simulink library "NeuroMuscularLibrary"  (R2019b)
settings: Solver=ode45  StartTime=0.0  StopTime=10.0  RelTol=1e-3  EnableMultiTasking=on
values from neighbouring files (symbols this model uses):
  a_18_19 = 116    [Prosthesis3R60Params.m]
  a_18_21 = 34    [Prosthesis3R60Params.m]
  a_2_3 = 18    [Prosthesis3R60Params.m]
  angle_offset = 0    [Prosthesis3R60Params.m]
  ankle_height = 0.08    [BodyMechParams.m]
  c = 0.05    [BodyMechParams.m]
  c_jointstop = 0.3 / (pi/180)    (= 17.1887338539)    [BodyMechParams.m]
  c_stance_comp_a0 = 885.0653    [Prosthesis3R60Params.m]
  c_stance_comp_a1 = 2.1443    [Prosthesis3R60Params.m]
  cg14 = 1/2*L14    (= 0.0475)    [Prosthesis3R60Params.m]
  cg25 = (5.45/11.05)*L25    (= 0.0379527149321)    [Prosthesis3R60Params.m]
  cg3 = (3.6/10.4)*L3    (= 0.0306346153846)    [Prosthesis3R60Params.m]
  d_fBall = 0.1    [BodyMechParams.m]
  d_fHeel = 0.05    [BodyMechParams.m]
  deltaLegAngleThr = 8*pi/180    (= 0.13962634016)    [CMGParams.m]
  DeltaThRef = 2e-3    (= 0.002)    [BodyMechParams.m]
  dt_visual = 0.001    [Prosthesis3R60Params.m]
  eref = 0.04    [BodyMechParams.m]
  Fmax = 4000    [MuscleEnergyTest.m]
  FmaxGLU = 1500    [BodyMechParams.m]
  footBallToAnkleDist = 0.16    [BodyMechParams.m]
  footBallToCenterDist = footLength/2    (= 0.1)    [BodyMechParams.m]
  footBallToHeelDist = footLength    (= 0.2)    [BodyMechParams.m]
  footCenterToCGDist = 0.14 - footBallToCenterDist    (= 0.04)    [BodyMechParams.m]
  footInertia = 0.005    [BodyMechParams.m]
  footLength = 0.2    [BodyMechParams.m]
  footMass = 1.25    [BodyMechParams.m]
  FT = 20    [MuscleEnergyTest.m]
  FT_GLU = 47.6    [BodyMechParams.m]
  g = 9.80665    [BodyMechParams.m]
  groundTheta = [atan(diff(groundZ)./diff(groundX)), 0]    [generateGround.m]
  groundZ = groundZ * stepSize/(largestStep+eps)    [generateGround.m]
  hatCenterToCGDist = 0.35 - hatHipToCenterDistLen    (= -0.05)    [BodyMechParams.m]
  hatHipToCenterDistLen = hatLength/2    (= 0.4)    [BodyMechParams.m]
  hatInertia = 3    [BodyMechParams.m]
  hatLeftHipToCenterDistWidth = .15    (= 0.15)    [BodyMechParams.m]
  hatLength = 0.8    [BodyMechParams.m]
  hatMass = 53.5    [BodyMechParams.m]
  hatThickness = 0.2    [BodyMechParams.m]
  hatWidth = 0.4    [BodyMechParams.m]
  J1011 = (4130)*1e-9    (= 4.13e-06)    [Prosthesis3R60Params.m]
  J1415 = (1.18*1e5)*1e-9    (= 0.000118)    [Prosthesis3R60Params.m]
  J18192021 = (6.86*1e4)*1e-9    (= 6.86e-05)    [Prosthesis3R60Params.m]
  J2526 = (3.59*1e4)*1e-9    (= 3.59e-05)    [Prosthesis3R60Params.m]
  J3467 = (25.96*1e4)*1e-9    (= 0.0002596)    [Prosthesis3R60Params.m]
  K = 5    [BodyMechParams.m]
  k_gn = k_gn/2    (= 39226.6)    [BodyMechParams.m]
  k_gt = k_gt/2    (= 39226.6)    [BodyMechParams.m]
  k_pressure = hatMass * g / DeltaThRef    (= 262327.8875)    [BodyMechParams.m]
  k_stance = 130000    [Prosthesis3R60Params.m]
  k_swing = 18750    [Prosthesis3R60Params.m]
  L0_stance = 0.08925    [Prosthesis3R60Params.m]
  L0_swing = 0.0896    [Prosthesis3R60Params.m]
  L10 = 7.9*1e-3    (= 0.0079)    [Prosthesis3R60Params.m]
  L11 = 3.3*1e-3    (= 0.0033)    [Prosthesis3R60Params.m]
  L14 = 95*1e-3    (= 0.095)    [Prosthesis3R60Params.m]
  L15 = 8.2*1e-3    (= 0.0082)    [Prosthesis3R60Params.m]
  L18 = 25.1*1e-3    (= 0.0251)    [Prosthesis3R60Params.m]
  L19 = 17.7*1e-3    (= 0.0177)    [Prosthesis3R60Params.m]
  L20 = 26*1e-3    (= 0.026)    [Prosthesis3R60Params.m]
  L21 = 1.7*1e-3    (= 0.0017)    [Prosthesis3R60Params.m]
  L25 = 76.95*1e-3    (= 0.07695)    [Prosthesis3R60Params.m]
  L26 = 2.8*1e-3    (= 0.0028)    [Prosthesis3R60Params.m]
  L3 = 88.5*1e-3    (= 0.0885)    [Prosthesis3R60Params.m]
  L4 = 1.7*1e-3    (= 0.0017)    [Prosthesis3R60Params.m]
  L6 = 40.25*1e-3    (= 0.04025)    [Prosthesis3R60Params.m]
  L7 = 14.9*1e-3    (= 0.0149)    [Prosthesis3R60Params.m]
  leg_l = [(thighLength - ankle_height/2) (shankLength - ankle_height/2)]    [BodyMechParams.m]
  legAngleSpeedMax = 10    [CMGParams.m]
  lopt = 0.055    [MuscleEnergyTest.m]
  loptBFSH = 0.12    [BodyMechParams.m]
  loptGAS = 0.05    [BodyMechParams.m]
  loptGLU = 0.11    [BodyMechParams.m]
  loptHAB = 0.09    [BodyMechParams.m]
  loptHAD = 0.10    (= 0.1)    [BodyMechParams.m]
  loptHAM = 0.10    (= 0.1)    [BodyMechParams.m]
  loptHFL = 0.11    [BodyMechParams.m]
  loptRF = 0.08    [BodyMechParams.m]
  loptSOL = 0.04    [BodyMechParams.m]
  loptTA = 0.06    [BodyMechParams.m]
  loptVAS = 0.08    [BodyMechParams.m]
  lslack = 0.245    [MuscleEnergyTest.m]
  lslackBFSH = 0.10    (= 0.1)    [BodyMechParams.m]
  lslackGAS = 0.40    (= 0.4)    [BodyMechParams.m]
  lslackGLU = 0.13    [BodyMechParams.m]
  lslackHAB = 0.07    [BodyMechParams.m]
  lslackHAD = 0.18    [BodyMechParams.m]
  lslackHAM = 0.31    [BodyMechParams.m]
  lslackHFL = 0.10    (= 0.1)    [BodyMechParams.m]
  lslackRF = 0.35    [BodyMechParams.m]
  lslackSOL = 0.26    [BodyMechParams.m]
  lslackTA = 0.24    [BodyMechParams.m]
  lslackVAS = 0.23    [BodyMechParams.m]
  m1011 = 49.5*1e-3    (= 0.0495)    [Prosthesis3R60Params.m]
  m1415 = 123.8*1e-3    (= 0.1238)    [Prosthesis3R60Params.m]
  m18192021 = 196.6*1e-3    (= 0.1966)    [Prosthesis3R60Params.m]
  m2526 = 58.3*1e-3    (= 0.0583)    [Prosthesis3R60Params.m]
  m3467 = 253.3*1e-3    (= 0.2533)    [Prosthesis3R60Params.m]
  mu_slide = 0.8    [BodyMechParams.m]
  mu_stick = 0.9    [BodyMechParams.m]
  N = 1.5    [BodyMechParams.m]    (also in cmaes.m = size(x,1); mergeCompareEnergyCosts.m = {S.name})
  phiKneeUpLimit = 5*pi/180    (= 0.0872664625997)    [BodyMechParams.m]
  phimaxGASa = (100-90)*pi/180    (= 0.174532925199)    [BodyMechParams.m]
  phimaxGASk = (180-140)*pi/180    (= 0.698131700798)    [BodyMechParams.m]
  phimaxRFk = (180-165)*pi/180    (= 0.261799387799)    [BodyMechParams.m]
  phimaxSOL = (100-90)*pi/180    (= 0.174532925199)    [BodyMechParams.m]
  phimaxTA = (80-90)*pi/180    (= -0.174532925199)    [BodyMechParams.m]
  phimaxVAS = (180-165)*pi/180    (= 0.261799387799)    [BodyMechParams.m]
  phirefBFSH = (180-160)*pi/180    (= 0.349065850399)    [BodyMechParams.m]
  phirefGASa = (80-90)*pi/180    (= -0.174532925199)    [BodyMechParams.m]
  phirefGASk = (180-165)*pi/180    (= 0.261799387799)    [BodyMechParams.m]
  phirefGLU = (120-180)*pi/180    (= -1.0471975512)    [BodyMechParams.m]
  phirefHAB = 10*pi/180    (= 0.174532925199)    [BodyMechParams.m]
  phirefHAD = 15*pi/180    (= 0.261799387799)    [BodyMechParams.m]
  phirefHAMh = (150-180)*pi/180    (= -0.523598775598)    [BodyMechParams.m]
  phirefHAMk = (180-180)*pi/180    (= 0)    [BodyMechParams.m]
  phirefHFL = (160-180)*pi/180    (= -0.349065850399)    [BodyMechParams.m]
  phirefRFh = (170-180)*pi/180    (= -0.174532925199)    [BodyMechParams.m]
  phirefRFk = (180-125)*pi/180    (= 0.959931088597)    [BodyMechParams.m]
  phirefSOL = (90-90)*pi/180    (= 0)    [BodyMechParams.m]
  ... (+64 more)
undefined symbols (not defined in the file or in its folder): ankleBackDriveGain, ankleCJointstop, ankleDgain, ankleFilterPID, ankleFilterSEA, ankleGearEff, ankleGearRatio, ankleIgain, ankleInitialAngle, ankleInputMass, ankleIntCoulomb, ankleIntDamping, ankleIntStatic, ankleParallelSpringDamping, ankleParallelSpringOffset, ankleParallelSpringStiffness, anklePgain, anklePlantarLimit, ankleSEADamping, ankleSEAStiffness, ankleTendonMass, ankleWMaxJointstop, D12_F, D12_S, D12_T, D12z_T, D13_F, D1G_F, D1G_HAT, D1G_S, D1G_T, D1Gy_F, DeltaS, DeltaSGLU, DeltaSHFL, dryFrictionDamping, dryFrictionStiffness, dryFrictionVelThresh, footMassp, FourBarL1, FourBarL3, GainDphiHATGLUst, GainDphiHATHABst, GainDphiHATHADst, GainDphiHATHFLst, GainFGASst, GainFGLUst, GainFHABst, GainFHAMst, GainFSOLst, GainFSOLTAst, GainFVASst, GainGAS, GainGLU, GainGLUswing, GainHAM, GainHAMHFL ... (+194)
libraries: sm_lib x332, nesl_utility x156, simulink x33, dspswit3 x30, $bdroot x19, simulink_extras x7
(part 3 of 15)

== system NeuroMuscularLibrary/HATs ==
  Brick Solid : sm_lib/Body Elements/Brick Solid  GraphicAmbientColor=[0.15 0.15 0.15 1.0]  BasedOnType=Mass  BrickDimensions=[L_HAT 0.1 2*D12z_T]  BrickDimensionUnits=m  CenterOfMass=[0 0 0]  CenterOfMassUnits=m  GraphicDiffuseColor=[0.5 0.5 0.5]  Density=0  DensityUnits=kg/m^3  DoExposeReferenceFrame=on  GraphicEmissiveColor=[0.0 0.0 0.0 1.0]  ExportEntireGeometry=off  SerializedFrames=<Frames/>  MarkerShape=Sphere  MarkerSize=10  GraphicType=FromGeometry  InertiaType=CalculateFromGeometry  Mass=0  MassUnits=kg  MomentsOfInertia=[1 1 1]  MomentsOfInertiaUnits=kg*m^2  GraphicOpacity=1.0  ProductsOfInertia=[0 0 0]  ProductsOfInertiaUnits=kg*m^2  GraphicShininess=75  GraphicSpecularColor=[0.5 0.5 0.5 1.0]  GraphicVisPropType=SimpleVisualProperties
  CS4 : sm_lib/Frames and Transforms/Rigid Transform  TranslationMethod=Cartesian  TranslationStandardOffset=0  TranslationLengthUnit=m  TranslationStandardAxis=+Z  TranslationCartesianOffset=[0 0 2*D12z_T]  TranslationROffset=0  TranslationROffsetUnits=m  TranslationZOffset=0  TranslationZOffsetUnits=m  TranslationThetaOffset=0  TranslationThetaOffsetUnits=deg  RotationMethod=None  RotationAngleUnits=deg  RotationStandardAxis=+Z  RotationAngle=0.0  RotationArbitraryAxis=[0 0 1]  FollAlignAxisA=+X  BaseAlignAxisA=+Y  FollAlignAxisB=+Y  BaseAlignAxisB=+Z  RotationSequenceAxes=FollowerAxes  RotationSequence=XYX  RotationSequenceAngles=[0 0 0]  RotationSequenceAnglesUnits=deg  RotationMatrix=[1 0 0; 0 1 0; 0 0 1]
  Inertia : sm_lib/Body Elements/Inertia  InertiaType=Custom  Mass=m_HAT  MassUnits=kg  CenterOfMass=[0 0 0]  CenterOfMassUnits=m  MomentsOfInertia="[Inx_HAT Iny_HAT  In_HAT]"  MomentsOfInertiaUnits=kg*m^2  ProductsOfInertia=[0 0 0]  ProductsOfInertiaUnits=kg*m^2  GraphicType=None  MarkerShape=Inertia  MarkerSize=20  GraphicVisPropType=SimpleVisualProperties  GraphicDiffuseColor=[0.5 0.5 0.5]  GraphicSpecularColor=[0.5 0.5 0.5 1.0]  GraphicAmbientColor=[0.15 0.15 0.15 1.0]  GraphicEmissiveColor=[0.0 0.0 0.0 1.0]  GraphicShininess=75  GraphicOpacity=1.0
  Mux{,1..5} (6 alike) : Mux  Inputs=3
  PS-Simulink Converter{,1..8} (9 alike) : nesl_utility/PS-Simulink Converter  PhysicalDomain=network_engine_domain  SubClassName=ps_output  LeftPortType=input  RightPortType=output  PseudoPeriodic=off  Frequencies=[]  Unit=m  AffineConversion=off
  PS-Simulink Converter{9..17} (9 alike) : nesl_utility/PS-Simulink Converter  PhysicalDomain=network_engine_domain  SubClassName=ps_output  LeftPortType=input  RightPortType=output  PseudoPeriodic=off  Frequencies=[]  Unit=m/s  AffineConversion=off
  Reference Frame : sm_lib/Frames and Transforms/Reference Frame
  TO: X-forward Y-up Z-lateral : sm_lib/Frames and Transforms/Rigid Transform  TranslationMethod=StandardAxis  TranslationStandardOffset=1*D12z_T/2  TranslationLengthUnit=m  TranslationStandardAxis=+Y  TranslationCartesianOffset=[0 0 0]  TranslationROffset=0  TranslationROffsetUnits=m  TranslationZOffset=0  TranslationZOffsetUnits=m  TranslationThetaOffset=0  TranslationThetaOffsetUnits=deg  RotationMethod=AlignedAxes  RotationAngleUnits=deg  RotationStandardAxis=+Z  RotationAngle=0  RotationArbitraryAxis=[0 0 1]  FollAlignAxisA=+Y  BaseAlignAxisA=+Z  FollAlignAxisB=+X  BaseAlignAxisB=+X  RotationSequenceAxes=FollowerAxes  RotationSequence=XYX  RotationSequenceAngles=[0 0 0]  RotationSequenceAnglesUnits=deg  RotationMatrix=[1 0 0; 0 1 0; 0 0 1]
  To CG : sm_lib/Frames and Transforms/Rigid Transform  TranslationMethod=Cartesian  TranslationStandardOffset=0  TranslationLengthUnit=m  TranslationStandardAxis=+Z  TranslationCartesianOffset=[D1G_HAT 0 D12z_T]  TranslationROffset=0  TranslationROffsetUnits=m  TranslationZOffset=0  TranslationZOffsetUnits=m  TranslationThetaOffset=0  TranslationThetaOffsetUnits=deg  RotationMethod=None  RotationAngleUnits=deg  RotationStandardAxis=+Z  RotationAngle=0.0  RotationArbitraryAxis=[0 0 1]  FollAlignAxisA=+X  BaseAlignAxisA=+Y  FollAlignAxisB=+Y  BaseAlignAxisB=+Z  RotationSequenceAxes=FollowerAxes  RotationSequence=XYX  RotationSequenceAngles=[0 0 0]  RotationSequenceAnglesUnits=deg  RotationMatrix=[1 0 0; 0 1 0; 0 0 1]
  To center : sm_lib/Frames and Transforms/Rigid Transform  TranslationMethod=Cartesian  TranslationStandardOffset=0  TranslationLengthUnit=m  TranslationStandardAxis=+Z  TranslationCartesianOffset=[L_HAT/2 0 D12z_T]  TranslationROffset=0  TranslationROffsetUnits=m  TranslationZOffset=0  TranslationZOffsetUnits=m  TranslationThetaOffset=0  TranslationThetaOffsetUnits=deg  RotationMethod=None  RotationAngleUnits=deg  RotationStandardAxis=+Z  RotationAngle=0.0  RotationArbitraryAxis=[0 0 1]  FollAlignAxisA=+Z  BaseAlignAxisA=-X  FollAlignAxisB=+Y  BaseAlignAxisB=+Y  RotationSequenceAxes=FollowerAxes  RotationSequence=XYX  RotationSequenceAngles=[0 0 0]  RotationSequenceAnglesUnits=deg  RotationMatrix=[1 0 0; 0 1 0; 0 0 1]
  Transform Sensor : sm_lib/Frames and Transforms/Transform Sensor  MeasurementFrame=NonRotatingBase  SenseAngle=off  SenseAxis=off  SenseAngle1=off  SenseAngle2=off  SenseAngle3=off  SenseQ=off  SenseR=off  SenseOmegaX=off  SenseOmegaY=off  SenseOmegaZ=off  SenseOmega1=off  SenseOmega2=off  SenseOmega3=off  SenseQDot=off  SenseRDot=off  SenseAlphaX=off  SenseAlphaY=off  SenseAlphaZ=off  SenseAlpha1=off  SenseAlpha2=off  SenseAlpha3=off  SenseQDDot=off  SenseRDDot=off  SenseX=on  SenseY=on  SenseZ=on  SenseRad=off  SenseAzim=off  SenseDist=off  SenseInc=off  SenseXDot=on  SenseYDot=on  SenseZDot=on  SenseRadDot=off  SenseAzimDot=off  SenseDistDot=off  SenseIncDot=off  SenseXDDot=off  SenseYDDot=off  SenseZDDot=off  SenseRadDDot=off  SenseAzimDDot=off  SenseDistDDot=off  SenseIncDDot=off
  Transform Sensor1 : sm_lib/Frames and Transforms/Transform Sensor  MeasurementFrame=NonRotatingBase  SenseAngle=off  SenseAxis=off  SenseAngle1=off  SenseAngle2=off  SenseAngle3=off  SenseQ=off  SenseR=off  SenseOmegaX=off  SenseOmegaY=off  SenseOmegaZ=off  SenseOmega1=off  SenseOmega2=off  SenseOmega3=off  SenseQDot=off  SenseRDot=off  SenseAlphaX=off  SenseAlphaY=off  SenseAlphaZ=off  SenseAlpha1=off  SenseAlpha2=off  SenseAlpha3=off  SenseQDDot=off  SenseRDDot=off  SenseX=on  SenseY=on  SenseZ=on  SenseRad=off  SenseAzim=off  SenseDist=off  SenseInc=off  SenseXDot=on  SenseYDot=on  SenseZDot=on  SenseRadDot=off  SenseAzimDot=off  SenseDistDot=off  SenseIncDot=off  SenseXDDot=off  SenseYDDot=off  SenseZDDot=off  SenseRadDDot=off  SenseAzimDDot=off  SenseDistDDot=off  SenseIncDDot=off
  Transform Sensor2 : sm_lib/Frames and Transforms/Transform Sensor  MeasurementFrame=NonRotatingBase  SenseAngle=off  SenseAxis=off  SenseAngle1=off  SenseAngle2=off  SenseAngle3=off  SenseQ=off  SenseR=off  SenseOmegaX=off  SenseOmegaY=off  SenseOmegaZ=off  SenseOmega1=off  SenseOmega2=off  SenseOmega3=off  SenseQDot=off  SenseRDot=off  SenseAlphaX=off  SenseAlphaY=off  SenseAlphaZ=off  SenseAlpha1=off  SenseAlpha2=off  SenseAlpha3=off  SenseQDDot=off  SenseRDDot=off  SenseX=on  SenseY=on  SenseZ=on  SenseRad=off  SenseAzim=off  SenseDist=off  SenseInc=off  SenseXDot=on  SenseYDot=on  SenseZDot=on  SenseRadDot=off  SenseAzimDot=off  SenseDistDot=off  SenseIncDot=off  SenseXDDot=off  SenseYDDot=off  SenseZDDot=off  SenseRadDDot=off  SenseAzimDDot=off  SenseDistDDot=off  SenseIncDDot=off
  World Frame1 : sm_lib/Frames and Transforms/World Frame
  Left hip : PMIOPort  Side=Left
  Right hip : PMIOPort  Port=2  Side=Left
  CG : PMIOPort  Port=3  Side=Right
  Left hip pos : Outport
  Left hip vel : Outport  Port=2
  HAT  pos : Outport  Port=3
  HAT  vel : Outport  Port=4
  Right hip pos : Outport  Port=5
  Right hip vel : Outport  Port=6
  wires:
  Mux/1 -> HAT  pos/1
  PS-Simulink Converter1/1 -> Mux/3
  PS-Simulink Converter2/1 -> Mux/2
  PS-Simulink Converter/1 -> Mux/1
  PS-Simulink Converter3/1 -> Mux1/1
  PS-Simulink Converter4/1 -> Mux1/2
  PS-Simulink Converter5/1 -> Mux1/3
  Mux2/1 -> Right hip pos/1
  PS-Simulink Converter8/1 -> Mux2/3
  PS-Simulink Converter7/1 -> Mux2/2
  PS-Simulink Converter6/1 -> Mux2/1
  Mux5/1 -> HAT  vel/1
  PS-Simulink Converter9/1 -> Mux5/1
  PS-Simulink Converter10/1 -> Mux5/2
  PS-Simulink Converter11/1 -> Mux5/3
  PS-Simulink Converter12/1 -> Mux3/1
  PS-Simulink Converter13/1 -> Mux3/2
  PS-Simulink Converter14/1 -> Mux3/3
  Mux3/1 -> Left hip vel/1
  PS-Simulink Converter15/1 -> Mux4/1
  PS-Simulink Converter16/1 -> Mux4/2
  PS-Simulink Converter17/1 -> Mux4/3
  Mux4/1 -> Right hip vel/1
  Mux1/1 -> Left hip pos/1
  connections:
  Reference Frame/RConn1 -- TO: X-forward Y-up Z-lateral/RConn1 -- Transform Sensor/LConn1 -- Transform Sensor2/LConn1 -- Transform Sensor1/LConn1
  Transform Sensor/RConn4 -- PS-Simulink Converter1/LConn1
  Transform Sensor/RConn3 -- PS-Simulink Converter2/LConn1
  PS-Simulink Converter/LConn1 -- Transform Sensor/RConn2
  Left hip/RConn1 -- Transform Sensor1/RConn1 -- CS4/LConn1 -- To CG/LConn1 -- To center/LConn1
  To CG/RConn1 -- CG/RConn1 -- Transform Sensor/RConn1 -- Inertia/RConn1
  Brick Solid/RConn1 -- To center/RConn1
  Right hip/RConn1 -- Transform Sensor2/RConn1 -- CS4/RConn1
  Transform Sensor1/RConn2 -- PS-Simulink Converter3/LConn1
  Transform Sensor1/RConn3 -- PS-Simulink Converter4/LConn1
  Transform Sensor1/RConn4 -- PS-Simulink Converter5/LConn1
  Transform Sensor2/RConn4 -- PS-Simulink Converter8/LConn1
  Transform Sensor2/RConn3 -- PS-Simulink Converter7/LConn1
  Transform Sensor2/RConn2 -- PS-Simulink Converter6/LConn1
  Transform Sensor/RConn7 -- PS-Simulink Converter11/LConn1
  Transform Sensor/RConn6 -- PS-Simulink Converter10/LConn1
  Transform Sensor/RConn5 -- PS-Simulink Converter9/LConn1
  Transform Sensor1/RConn5 -- PS-Simulink Converter12/LConn1
  Transform Sensor1/RConn6 -- PS-Simulink Converter13/LConn1
  Transform Sensor1/RConn7 -- PS-Simulink Converter14/LConn1
  Transform Sensor2/RConn5 -- PS-Simulink Converter15/LConn1
  Transform Sensor2/RConn6 -- PS-Simulink Converter16/LConn1
  Transform Sensor2/RConn7 -- PS-Simulink Converter17/LConn1
  TO: X-forward Y-up Z-lateral/LConn1 -- World Frame1/RConn1

== system NeuroMuscularLibrary/HFL Link ==
  note: HFL Attachment
  hip angle [rad] : Inport
  Constant : Constant  Value=lslackHFL+loptHFL
  Constant1 : Constant  Value=rHFL
  Constant2 : Constant  Value=phirefHFL
  Gain2 : Gain  Gain=rhoHFL
  Product : Product  RndMeth=Zero
  Sum2 : Sum  Inputs=|+-
  Sum5 : Sum  Inputs=|++
  lmtu [m] : Outport
  lever [m] : Outport  Port=2
  wires:
  Constant/1 -> Sum5/1
  Sum5/1 -> lmtu [m]/1
  Product/1 -> Gain2/1
  Constant2/1 -> Sum2/2
  Sum2/1 -> Product/1
  Constant1/1 -> Product/2, lever [m]/1
  Gain2/1 -> Sum5/2
  hip angle [rad]/1 -> Sum2/1

== system NeuroMuscularLibrary/Hard Stops ==
  Muscle Torques : Inport
  phiANDdphiHip : Inport  Port=2
  phiANDdphiKnee : Inport  Port=3
  phiANDdphiAnkle : Inport  Port=4
  Muscle Torques R : Inport  Port=5
  phiANDdphiHipR : Inport  Port=6
  Add : Sum
  Add1 : Sum
  Ankle Joint Limit : $bdroot/Overextension//Overflexion Joint Limit  phiUpLimit=phi12_UpLimit  phiLowLimit=phi12_LowLimit
  Demux{,1..3} (4 alike) : Demux  Outputs=2
  Hip Overextension Joint Limit : $bdroot/Overextension Joint Limit  phiUpLimit=phi34_UpLimit  ext=1
  Knee Overextension Joint Limit : $bdroot/Overextension Joint Limit  phiUpLimit=phi23_UpLimit  ext=1
  L Hip Roll Joint Limits : Subsystem
  Mux : Mux  Inputs=3
  Net Torque : Outport
  Hip Stop Torque : Outport  Port=2
  Knee Stop Torque : Outport  Port=3
  Ankle Stop Torque : Outport  Port=4
  Net Torque R : Outport  Port=5
  Hip R Stop Torque : Outport  Port=6
  wires:
  Knee Overextension Joint Limit/1 -> Knee Stop Torque/1, Mux/2
  Muscle Torques/1 -> Add/1
  Mux/1 -> Add/2
  Ankle Joint Limit/1 -> Ankle Stop Torque/1, Mux/3
  Demux/2 -> Knee Overextension Joint Limit/2
  Demux/1 -> Knee Overextension Joint Limit/1
  Demux1/1 -> Hip Overextension Joint Limit/1
  Demux1/2 -> Hip Overextension Joint Limit/2
  Demux2/1 -> Ankle Joint Limit/1
  Demux2/2 -> Ankle Joint Limit/2
  phiANDdphiKnee/1 -> Demux/1
  Hip Overextension Joint Limit/1 -> Hip Stop Torque/1, Mux/1
  phiANDdphiHip/1 -> Demux1/1
  phiANDdphiAnkle/1 -> Demux2/1
  Add/1 -> Net Torque/1
  Demux3/2 -> L Hip Roll Joint Limits/2(dphi [rad/s])
  Demux3/1 -> L Hip Roll Joint Limits/1(phi [rad])
  phiANDdphiHipR/1 -> Demux3/1
  Add1/1 -> Net Torque R/1
  L Hip Roll Joint Limits/1(M_stop [Nm]) -> Hip R Stop Torque/1, Add1/2
  Muscle Torques R/1 -> Add1/1

== system NeuroMuscularLibrary/Hill Muscle ==
  note: Excitation Contraction Coupling
  note: Muscle-Tendon Dynamics
  STIM : Inport
  lmtc [m] : Inport  Port=2
  1 : Product  Inputs=**  SaturateOnIntegerOverflow=on  InputSameDT=on  OutDataTypeStr=Inherit: Same as first input
  1/lslack : Gain  Gain=1/lslack  SaturateOnIntegerOverflow=on  OutDataTypeStr=Inherit: Same as input  ParamDataTypeStr=Inherit: Same as input
  Add : Sum  Inputs=+-
  BE force-length relation : Subsystem
  CE force-length relation : Subsystem
  CE inverse force-velocity relation : Subsystem
  Constant : Constant  Value=lslack
  ECC TransferFcn : simulink_extras/Additional Linear/Transfer Fcn (with initial outputs)  N=[1]  D="[tau  1]"  Y0=preA  U0=0
      settings: AttributesFormatString=pre-activation: %<Y0>
  Fmax : Gain  Gain=Fmax  SaturateOnIntegerOverflow=on  OutDataTypeStr=Inherit: Same as input  ParamDataTypeStr=Inherit: Same as input
  Fv = Fse / (A*Fce) : Product  Inputs=*/  SaturateOnIntegerOverflow=on  InputSameDT=on  OutDataTypeStr=Inherit: Same as first input
  Integrator : Integrator  InitialConditionSource=external  LowerSaturationLimit=0.05
  PE force-length relation : Subsystem
  SE force-length relation : Subsystem
  Sum : Sum  Inputs=|+-  SaturateOnIntegerOverflow=on  InputSameDT=on  OutDataTypeStr=Inherit: Same as first input
  Sum2 : Sum  Inputs=|-+  SaturateOnIntegerOverflow=on  InputSameDT=on  OutDataTypeStr=Inherit: Same as first input
  Sum3 : Sum  SaturateOnIntegerOverflow=on  InputSameDT=on  OutDataTypeStr=Inherit: Same as first input
  Sum4 : Sum  SaturateOnIntegerOverflow=on  InputSameDT=on  OutDataTypeStr=Inherit: Same as first input
  lce/lopt : Gain  Gain=1/lopt  SaturateOnIntegerOverflow=on  OutDataTypeStr=Inherit: Same as input  ParamDataTypeStr=Inherit: Same as input
  lce/lopt1 : Gain  Gain=1/lopt  SaturateOnIntegerOverflow=on  OutDataTypeStr=Inherit: Same as input  ParamDataTypeStr=Inherit: Same as input
  lopt : Gain  Gain=lopt  SaturateOnIntegerOverflow=on  OutDataTypeStr=Inherit: Same as input  ParamDataTypeStr=Inherit: Same as input
  vmax : Gain  Gain=vmax  SaturateOnIntegerOverflow=on  OutDataTypeStr=Inherit: Same as input  ParamDataTypeStr=Inherit: Same as input
  Fmtc : Outport  InitialOutput=0
  Lce [lopt] : Outport  Port=2  InitialOutput=0
  Vce [lopt] : Outport  Port=3  InitialOutput=0
  Lse : Outport  Port=4  InitialOutput=0
  A : Outport  Port=5  InitialOutput=0
  fce : Outport  Port=6
  wires:
  ECC TransferFcn/1 -> 1/2, A/1
  STIM/1 -> ECC TransferFcn/1
  CE inverse force-velocity relation/1(v[vmax]) -> vmax/1
  Sum3/1 -> Fv = Fse / (A*Fce)/2
  BE force-length relation/1(fbe [Fmax]) -> Sum4/2
  1/1 -> Sum3/2
  PE force-length relation/1(fpe [Fmax]) -> Sum3/1, Add/2
  Sum4/1 -> Add/1, Fv = Fse / (A*Fce)/1  "fse+fbe"
  CE force-length relation/1(fce [Fmax]) -> 1/1  "f_l"
  Constant/1 -> Sum2/1
  Sum2/1 -> Integrator/2
  SE force-length relation/1(fse [Fmax]) -> Sum4/1, Fmax/1
  1/lslack/1 -> SE force-length relation/1(lse [lslack])
  Fmax/1 -> Fmtc/1  "Fmtc"
  lmtc [m]/1 -> Sum/1, Sum2/2  "lmtc"
  vmax/1 -> lopt/1, Vce [lopt]/1  "vce"
  Fv = Fse / (A*Fce)/1 -> CE inverse force-velocity relation/1(Fv[Fmax])  "fv"
  lce/lopt/1 -> PE force-length relation/1(lce [lopt]), BE force-length relation/1(lce [lopt]), CE force-length relation/1(lce [lopt])
  Sum/1 -> Lse/1, 1/lslack/1  "lse"
  Integrator/1 -> lce/lopt1/1, lce/lopt/1, Sum/2  "lce"
  Add/1 -> fce/1
  lce/lopt1/1 -> Lce [lopt]/1
  lopt/1 -> Integrator/1  "vce"

== system NeuroMuscularLibrary/Leg Angle//Length ==
  Constant : Constant  Value=pi
  Demux : Demux  Outputs=2
  Mux : Mux  Inputs=3
  Mux1 : Mux  Inputs=3
  PS-Simulink Converter{,1..6} (7 alike) : nesl_utility/PS-Simulink Converter  PhysicalDomain=network_engine_domain  SubClassName=ps_output  LeftPortType=input  RightPortType=output  PseudoPeriodic=off  Frequencies=[]  Unit=m  AffineConversion=off
  Position Sensor : sm_lib/Frames and Transforms/Transform Sensor  MeasurementFrame=World  SenseAngle=off  SenseAxis=off  SenseAngle1=off  SenseAngle2=off  SenseAngle3=off  SenseQ=off  SenseR=off  SenseOmegaX=off  SenseOmegaY=off  SenseOmegaZ=off  SenseOmega1=off  SenseOmega2=off  SenseOmega3=off  SenseQDot=off  SenseRDot=off  SenseAlphaX=off  SenseAlphaY=off  SenseAlphaZ=off  SenseAlpha1=off  SenseAlpha2=off  SenseAlpha3=off  SenseQDDot=off  SenseRDDot=off  SenseX=on  SenseY=on  SenseZ=on  SenseRad=off  SenseAzim=off  SenseDist=off  SenseInc=off  SenseXDot=off  SenseYDot=off  SenseZDot=off  SenseRadDot=off  SenseAzimDot=off  SenseDistDot=off  SenseIncDot=off  SenseXDDot=off  SenseYDDot=off  SenseZDDot=off  SenseRadDDot=off  SenseAzimDDot=off  SenseDistDDot=off  SenseIncDDot=off
  Position Sensor1 : sm_lib/Frames and Transforms/Transform Sensor  MeasurementFrame=World  SenseAngle=off  SenseAxis=off  SenseAngle1=off  SenseAngle2=off  SenseAngle3=off  SenseQ=off  SenseR=off  SenseOmegaX=off  SenseOmegaY=off  SenseOmegaZ=off  SenseOmega1=off  SenseOmega2=off  SenseOmega3=off  SenseQDot=off  SenseRDot=off  SenseAlphaX=off  SenseAlphaY=off  SenseAlphaZ=off  SenseAlpha1=off  SenseAlpha2=off  SenseAlpha3=off  SenseQDDot=off  SenseRDDot=off  SenseX=on  SenseY=on  SenseZ=on  SenseRad=off  SenseAzim=off  SenseDist=off  SenseInc=off  SenseXDot=off  SenseYDot=off  SenseZDot=off  SenseRadDot=off  SenseAzimDot=off  SenseDistDot=off  SenseIncDot=off  SenseXDDot=off  SenseYDDot=off  SenseZDDot=off  SenseRadDDot=off  SenseAzimDDot=off  SenseDistDDot=off  SenseIncDDot=off
  Selector : Selector  InputPortWidth=3  IndexOptions=Index vector (dialog)  Indices=[3 1]  OutputSizes=1
  Subtract : Sum  Inputs=+-
  Sum : Sum  Inputs=|-+
  Transform Sensor : sm_lib/Frames and Transforms/Transform Sensor  MeasurementFrame=World  SenseAngle=off  SenseAxis=off  SenseAngle1=off  SenseAngle2=off  SenseAngle3=off  SenseQ=off  SenseR=off  SenseOmegaX=off  SenseOmegaY=off  SenseOmegaZ=off  SenseOmega1=off  SenseOmega2=off  SenseOmega3=off  SenseQDot=off  SenseRDot=off  SenseAlphaX=off  SenseAlphaY=off  SenseAlphaZ=off  SenseAlpha1=off  SenseAlpha2=off  SenseAlpha3=off  SenseQDDot=off  SenseRDDot=off  SenseX=off  SenseY=off  SenseZ=off  SenseRad=off  SenseAzim=off  SenseDist=on  SenseInc=off  SenseXDot=off  SenseYDot=off  SenseZDot=off  SenseRadDot=off  SenseAzimDot=off  SenseDistDot=off  SenseIncDot=off  SenseXDDot=off  SenseYDDot=off  SenseZDDot=off  SenseRadDDot=off  SenseAzimDDot=off  SenseDistDDot=off  SenseIncDDot=off
  Trigonometric Function : Trigonometry  Operator=atan2  OutputSignalType=real
  World Frame : sm_lib/Frames and Transforms/World Frame
  Hip : PMIOPort  Side=Left
  Ankle : PMIOPort  Port=2  Side=Left
  Leg Angle : Outport
  Leg Length : Outport  Port=2
  wires:
  PS-Simulink Converter6/1 -> Leg Length/1
  PS-Simulink Converter2/1 -> Mux/3
  PS-Simulink Converter/1 -> Mux/1
  PS-Simulink Converter1/1 -> Mux/2
  PS-Simulink Converter5/1 -> Mux1/3
  PS-Simulink Converter3/1 -> Mux1/1
  PS-Simulink Converter4/1 -> Mux1/2
  Mux/1 -> Subtract/1
  Mux1/1 -> Subtract/2
  Trigonometric Function/1 -> Sum/1
  Sum/1 -> Leg Angle/1
  Constant/1 -> Sum/2
  Subtract/1 -> Selector/1
  Selector/1 -> Demux/1
  Demux/1 -> Trigonometric Function/1
  Demux/2 -> Trigonometric Function/2
  connections:
  PS-Simulink Converter6/LConn1 -- Transform Sensor/RConn2
  PS-Simulink Converter2/LConn1 -- Position Sensor/RConn4
  PS-Simulink Converter/LConn1 -- Position Sensor/RConn2
  Transform Sensor/RConn1 -- Hip/RConn1 -- Position Sensor/RConn1
  PS-Simulink Converter1/LConn1 -- Position Sensor/RConn3
  World Frame/RConn1 -- Position Sensor/LConn1 -- Position Sensor1/LConn1
  PS-Simulink Converter4/LConn1 -- Position Sensor1/RConn3
  PS-Simulink Converter5/LConn1 -- Position Sensor1/RConn4
  PS-Simulink Converter3/LConn1 -- Position Sensor1/RConn2
  Transform Sensor/LConn1 -- Ankle/RConn1 -- Position Sensor1/RConn1

== system NeuroMuscularLibrary/Leg step length//vel calculator ==
  Hip x pos : Inport
  Simulation time : Inport  Port=2
  Enable : EnablePort
  Difference : simulink/Discrete/Difference  ICPrevInput=0.0  OutMin=[]  OutMax=[]  OutDataType=fixdt(1, 16)  OutScaling=2^-10  DoSatur=off
  Difference1 : simulink/Discrete/Difference  ICPrevInput=0.0  OutMin=[]  OutMax=[]  OutDataType=fixdt(1, 16)  OutScaling=2^-10  DoSatur=off
  Divide : Product  Inputs=*/
  Step length : Outport  OutputWhenDisabled=reset  InitialOutput=[0]
  Step time : Outport  Port=2  OutputWhenDisabled=reset  InitialOutput=[0]
  Step avg velocity : Outport  Port=3  OutputWhenDisabled=reset  InitialOutput=[0]
  wires:
  Hip x pos/1 -> Difference/1
  Difference/1 -> Divide/1, Step length/1
  Simulation time/1 -> Difference1/1
  Difference1/1 -> Divide/2, Step time/1
  Divide/1 -> Step avg velocity/1

== system NeuroMuscularLibrary/Lower Thigh ==
  Knee Solid : sm_lib/Body Elements/Cylindrical Solid  GraphicAmbientColor=[0.15 0.15 0.15 1.0]  BasedOnType=Density  CenterOfMass=[0 0 thighCenterToCGDist*ThPos]  CenterOfMassUnits=m  GraphicDiffuseColor=[0.5 0.5 0.5]  CylinderLength=thighLength*ThPos  CylinderLengthUnits=m  CylinderRadius=.075  CylinderRadiusUnits=m  Density=1000  DensityUnits=kg/(m^3)  DoExposeReferenceFrame=on  GraphicEmissiveColor=[0.0 0.0 0.0 1.0]  ExportEntireGeometry=off  SerializedFrames=<Frames/>  MarkerShape=Sphere  MarkerSize=10  GraphicType=FromGeometry  InertiaType=Custom  Mass=thighMass*ThPos  MassUnits=kg  MomentsOfInertia=[thighInertia*(ThPos)^3 0 0]  MomentsOfInertiaUnits=kg*m^2  GraphicOpacity=1.0  ProductsOfInertia=[0 0 0]  ProductsOfInertiaUnits=kg*m^2  GraphicShininess=75  GraphicSpecularColor=[0.5 0.5 0.5 1.0]  GraphicVisPropType=SimpleVisualProperties
  Knee to Center : sm_lib/Frames and Transforms/Rigid Transform  TranslationMethod=Cartesian  TranslationStandardOffset=0  TranslationLengthUnit=m  TranslationStandardAxis=+Z  TranslationCartesianOffset=[0 thighKneeToCenterDist*ThPos 0]  TranslationROffset=0  TranslationROffsetUnits=m  TranslationZOffset=0  TranslationZOffsetUnits=m  TranslationThetaOffset=0  TranslationThetaOffsetUnits=deg  RotationMethod=AlignedAxes  RotationAngleUnits=deg  RotationStandardAxis=+Z  RotationAngle=0  RotationArbitraryAxis=[0 0 1]  FollAlignAxisA=+Z  BaseAlignAxisA=+Y  FollAlignAxisB=+X  BaseAlignAxisB=+X  RotationSequenceAxes=FollowerAxes  RotationSequence=XYX  RotationSequenceAngles=[0 0 0]  RotationSequenceAnglesUnits=deg  RotationMatrix=[1 0 0; 0 1 0; 0 0 1]
  Knee to Sensor Sheet : sm_lib/Frames and Transforms/Rigid Transform  TranslationMethod=Cartesian  TranslationStandardOffset=0  TranslationLengthUnit=m  TranslationStandardAxis=+Z  TranslationCartesianOffset=[0 thighKneeToHipDist*ThPos 0]  TranslationROffset=0  TranslationROffsetUnits=m  TranslationZOffset=0  TranslationZOffsetUnits=m  TranslationThetaOffset=0  TranslationThetaOffsetUnits=deg  RotationMethod=None  RotationAngleUnits=deg  RotationStandardAxis=+Z  RotationAngle=0  RotationArbitraryAxis=[0 0 1]  FollAlignAxisA=+Z  BaseAlignAxisA=+X  FollAlignAxisB=+Y  BaseAlignAxisB=+Y  RotationSequenceAxes=FollowerAxes  RotationSequence=XYX  RotationSequenceAngles=[0 0 0]  RotationSequenceAnglesUnits=deg  RotationMatrix=[1 0 0; 0 1 0; 0 0 1]
  Thigh CG : sm_lib/Frames and Transforms/Reference Frame
  Thigh Center to CG : sm_lib/Frames and Transforms/Rigid Transform  TranslationMethod=Cartesian  TranslationStandardOffset=0  TranslationLengthUnit=m  TranslationStandardAxis=+Z  TranslationCartesianOffset=[0 0 thighCenterToCGDist*ThPos]  TranslationROffset=0  TranslationROffsetUnits=m  TranslationZOffset=0  TranslationZOffsetUnits=m  TranslationThetaOffset=0  TranslationThetaOffsetUnits=deg  RotationMethod=None  RotationAngleUnits=deg  RotationStandardAxis=+Z  RotationAngle=0  RotationArbitraryAxis=[0 0 1]  FollAlignAxisA=+X  BaseAlignAxisA=+Y  FollAlignAxisB=+Y  BaseAlignAxisB=+Z  RotationSequenceAxes=FollowerAxes  RotationSequence=XYX  RotationSequenceAngles=[0 0 0]  RotationSequenceAnglesUnits=deg  RotationMatrix=[1 0 0; 0 1 0; 0 0 1]
  Knee : PMIOPort  Side=Left
  Sensor Sheet : PMIOPort  Port=2  Side=Right
  connections:
  Knee/RConn1 -- Knee to Center/LConn1 -- Knee to Sensor Sheet/LConn1
  Knee to Center/RConn1 -- Knee Solid/RConn1 -- Thigh Center to CG/LConn1
  Knee to Sensor Sheet/RConn1 -- Sensor Sheet/RConn1
  Thigh Center to CG/RConn1 -- Thigh CG/RConn1

== system NeuroMuscularLibrary/Muscle Energy ==
  Dynamics : Inport
  Stimulation : Inport  Port=2
  Muscle Energy Umberger (2003) : $bdroot/Muscle Energy Umberger (2003)  lopt=lopt  FT=FT  Fmax=Fmax  vmax=vmax
  Muscle Energy Umberger (2003) TG : $bdroot/Muscle Energy Umberger (2003) TG  lopt=lopt  FT=FT  Fmax=Fmax
  Muscle Energy Umberger (2010) : $bdroot/Muscle Energy Umberger (2010)  lopt=lopt  FT=FT  Fmax=Fmax  vmax=vmax
  Muscle Energy Wang (2012) : $bdroot/Muscle Energy Wang (2012)  lopt=lopt  FT=FT  Fmax=Fmax
  Mux : Mux
  Power : Outport
  wires:
  Dynamics/1 -> Muscle Energy Umberger (2010)/1, Muscle Energy Umberger (2003) TG/1, Muscle Energy Umberger (2003)/1, Muscle Energy Wang (2012)/1
  Stimulation/1 -> Muscle Energy Umberger (2003)/2, Muscle Energy Umberger (2003) TG/2, Muscle Energy Wang (2012)/2, Muscle Energy Umberger (2010)/2
  Mux/1 -> Power/1
  Muscle Energy Umberger (2003)/1 -> Mux/1
  Muscle Energy Umberger (2003) TG/1 -> Mux/2
  Muscle Energy Umberger (2010)/1 -> Mux/3
  Muscle Energy Wang (2012)/1 -> Mux/4

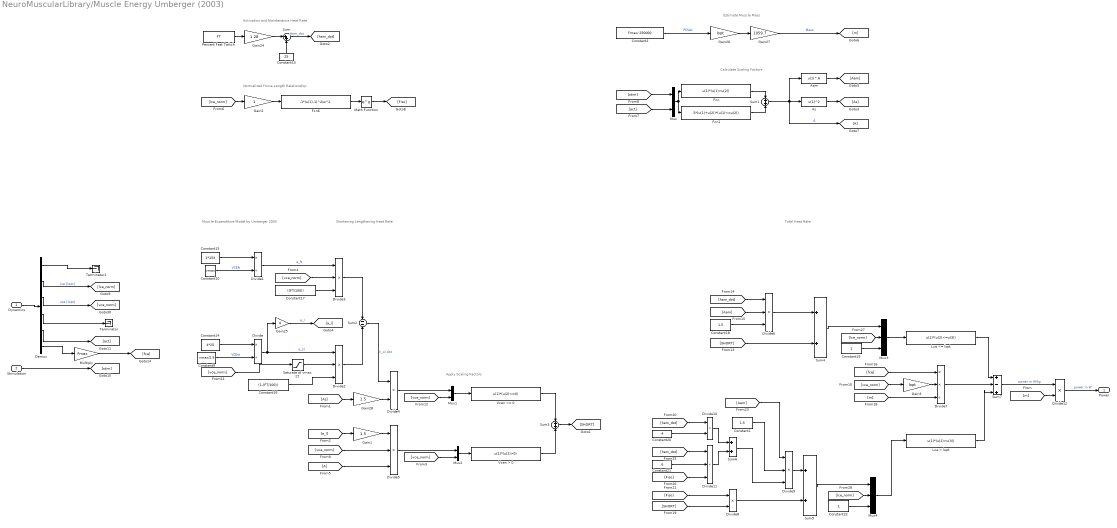
== system NeuroMuscularLibrary/Muscle Energy Umberger (2003) ==
  note: Muscle Expenditure Model by Umberger 2003
  note: Total Heat Rate
  note: Estimate Muscle Mass
  note: Calculate Scaling Factors
  note: Apply Scaling Factors
  note: Shortening Lengthening Heat Rate
  note: Normalized Force-Length Relationship
  note: Activation and Maintenance Heat Rate
  Dynamics : Inport
  Stimulation : Inport  Port=2
  "Aam " : Fcn  Expr=u(1)^.6
  As : Fcn  Expr=u(1)^2
  Constant1 : Constant  Value=1.5
  Constant10 : Constant  Value=vmax
  Constant13 : Constant  Value=25
  Constant14 : Constant  Value=4*25
  Constant15 : Constant  Value=1*153
  Constant16 : Constant  Value=(1-(FT/100))
  Constant17 : Constant  Value=((FT/100))
  Constant18 : Constant  Value=1.5
  Constant19 : Constant
  Constant2 : Constant  Value=Fmax/ 250000
  Constant20 : Constant  Value=.4
  Constant21 : Constant  Value=.6
  Constant22 : Constant
  Constant9 : Constant  Value=vmax/2.5
  Demux : Demux  Outputs=6
  Divide : Product  Inputs=*/
  Divide1 : Product  Inputs=*/
  Divide{4,8,10,12} (4 alike) : Product  Inputs=**
  Divide{2..3,5..6,9,11} (6 alike) : Product  Inputs=***
  Divide7 : Product  Inputs=**/
  Fcn : Fcn  Expr=u(1)*(u(1)>u(2))
  Fcn1 : Fcn  Expr=.5*(u(1)+u(2))*(u(1)<=u(2))
  Fcn6 : Fcn  Expr=-1*(u(1)-1)^2/w^2
  Gain1 : Gain  Gain=1.5
  Gain2 : Gain
  Gain24 : Gain  Gain=1.28
  Gain25 : Gain  Gain=4
  Gain26 : Gain  Gain=lopt
  Gain27 : Gain  Gain=1059.7
  Gain28 : Gain  Gain=1.5
  Gain3 : Gain  Gain=lopt
  Lce <= lopt : Fcn  Expr=u(1)*(u(2)<=u(3))
  Lce > lopt : Fcn  Expr=u(1)*(u(2)>u(3))
  Math Function : Math  SaturateOnIntegerOverflow=on
  Multiply : Gain  Gain=Fmax
  Mux : Mux  Inputs=2
  Mux1 : Mux  Inputs=2
  Mux2 : Mux  Inputs=2
  Mux3 : Mux  Inputs=3
  Mux4 : Mux  Inputs=3
  Percent Fast Twitch : Constant  Value=FT
  Saturate at vmax ST : Saturate  UpperLimit=vmax/2.5  LowerLimit=-vmax/2.5  ZeroCross=off
  Sum : Sum  Inputs=|++
  Sum1 : Sum  Inputs=+|+
  Sum2 : Sum  Inputs=-|-
  Sum3 : Sum  Inputs=+|+
  Sum4 : Sum
  Sum5 : Sum
  Sum6 : Sum
  Sum7 : Sum  Inputs=+-+
  Terminator : Terminator
  Terminator1 : Terminator
  "Vcen <= 0 " : Fcn  Expr=u(1)*(u(2)<=0)
  Vcen > 0 : Fcn  Expr=u(1)*(u(2)>0)
  Power : Outport
  wires:
  Demux/6 -> Multiply/1
  Gain2/1 -> Fcn6/1
  [lce_norm] -> Gain2/1
  Demux/4 -> Terminator/1
  Demux/5 -> [act]
  Demux/3 -> [vce_norm]  "vce [lopt]"
  Demux/2 -> [lce_norm]  "lce [lopt]"
  Demux/1 -> Terminator1/1
  Stimulation/1 -> [stim]
  Dynamics/1 -> Demux/1
  [As] -> Gain28/1
  "Vcen <= 0 "/1 -> Sum3/1
  Sum3/1 -> [SHORT]
  Mux2/1 -> Vcen > 0/1
  Gain27/1 -> [m]  "Mass"
  Constant9/1 -> Divide/2  "VCEst"
  Gain28/1 -> Divide4/2
  [lce_norm] -> Mux3/2
  Mux3/1 -> Lce <= lopt/1
  [SHORT] -> Divide8/2
  Constant2/1 -> Gain26/1  "PCSAL"
  Constant21/1 -> Divide11/2
  [vce_norm] -> Mux2/2
  Percent Fast Twitch/1 -> Gain24/1
  Mux/1 -> Fcn/1, Fcn1/1
  Sum/1 -> [ham_dot]  "Ham_dot"
  Sum2/1 -> Divide4/1  "h_sl dot"
  Constant20/1 -> Divide10/2
  As/1 -> [As]
  Divide8/1 -> Sum5/2
  Constant13/1 -> Sum/2
  Fcn/1 -> Sum1/1
  Fcn1/1 -> Sum1/2
  [vce_norm] -> Divide3/2
  Mux1/1 -> "Vcen <= 0 "/1
  Divide4/1 -> Mux1/1
  Constant15/1 -> Divide1/1
  Constant18/1 -> Divide6/3
  Sum1/1 -> [A], As/1, "Aam "/1  "A"
  [ham_dot] -> Divide6/1
  Divide/1 -> Divide2/1, Gain25/1  "a_st"
  Divide6/1 -> Sum4/1
  Constant14/1 -> Divide/1
  Divide5/1 -> Mux2/1
  Constant22/1 -> Mux4/3
  Vcen > 0/1 -> Sum3/2
  Sum7/1 -> Divide12/1  "power in W/kg"
  [vce_norm] -> Mux1/2
  Divide1/1 -> Divide3/1  "a_ft"
  [vce_norm] -> Saturate at vmax ST/1
  Divide2/1 -> Sum2/2
  Constant10/1 -> Divide1/2  "VCEft"
  "Aam "/1 -> [Aam]
  Math Function/1 -> [Fiso]
  Gain25/1 -> [a_l]  "a_l"
  Divide3/1 -> Sum2/1
  [Fiso] -> Divide11/3
  Constant17/1 -> Divide3/3
  Constant16/1 -> Divide2/3
  Gain1/1 -> Divide5/1
  [Aam] -> Divide6/2
  [a_l] -> Gain1/1
  [vce_norm] -> Divide5/2
  Mux4/1 -> Lce > lopt/1
  Constant19/1 -> Mux3/3
  [SHORT] -> Sum4/2
  Sum6/1 -> Divide9/3
  Sum5/1 -> Mux4/1
  [ham_dot] -> Divide10/1
  [lce_norm] -> Mux4/2
  Divide11/1 -> Sum6/2
  [ham_dot] -> Divide11/1
  [A] -> Divide5/3
  Fcn6/1 -> Math Function/1
  [Fiso] -> Divide8/1
  Divide12/1 -> Power/1  "power in W"
  Sum4/1 -> Mux3/1
  Divide10/1 -> Sum6/1
  Gain24/1 -> Sum/1
  Gain26/1 -> Gain27/1
  [stim] -> Mux/1
  [act] -> Mux/2
  Divide7/1 -> Sum7/2
  [vce_norm] -> Gain3/1
  [fce] -> Divide7/1
  [m] -> Divide7/3
  Constant1/1 -> Divide9/2
  [Aam] -> Divide9/1
  Divide9/1 -> Sum5/1
  [m] -> Divide12/2
  Saturate at vmax ST/1 -> Divide2/2
  Multiply/1 -> [fce]
  Lce <= lopt/1 -> Sum7/1
  Lce > lopt/1 -> Sum7/3
  Gain3/1 -> Divide7/2

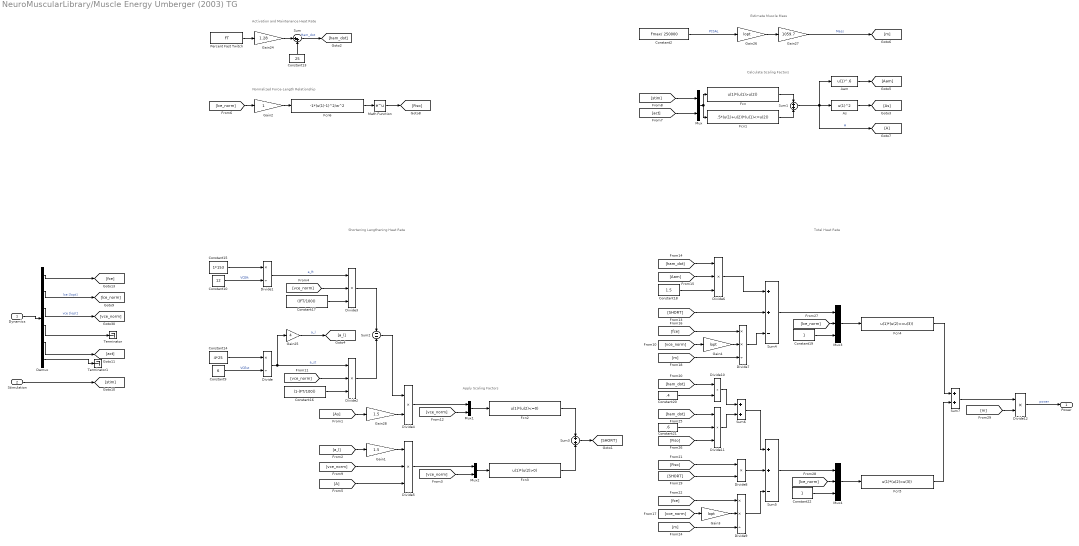
== system NeuroMuscularLibrary/Muscle Energy Umberger (2003) TG ==
  note: Activation and Maintenance Heat Rate
  note: Normalized Force-Length Relationship
  note: Shortening Lengthening Heat Rate
  note: Apply Scaling Factors
  note: Calculate Scaling Factors
  note: Estimate Muscle Mass
  note: Total Heat Rate
  Dynamics : Inport
  Stimulation : Inport  Port=2
  "Aam " : Fcn  Expr=u(1)^.6
  As : Fcn  Expr=u(1)^2
  Constant10 : Constant  Value=12
  Constant13 : Constant  Value=25
  Constant14 : Constant  Value=4*25
  Constant15 : Constant  Value=1*153
  Constant16 : Constant  Value=(1-(FT/100))
  Constant17 : Constant  Value=((FT/100))
  Constant18 : Constant  Value=1.5
  Constant19 : Constant
  Constant2 : Constant  Value=Fmax/ 250000
  Constant20 : Constant  Value=.4
  Constant21 : Constant  Value=.6
  Constant22 : Constant
  Constant9 : Constant  Value=6
  Demux : Demux  Outputs=6
  Divide : Product  Inputs=*/
  Divide1 : Product  Inputs=*/
  Divide{4,8,10,12} (4 alike) : Product  Inputs=**
  Divide{2..3,5..6,11} (5 alike) : Product  Inputs=***
  Divide7 : Product  Inputs=**/
  Divide9 : Product  Inputs=**/
  Fcn : Fcn  Expr=u(1)*(u(1)>u(2))
  Fcn1 : Fcn  Expr=.5*(u(1)+u(2))*(u(1)<=u(2))
  Fcn2 : Fcn  Expr=u(1)*(u(2)<=0)
  Fcn3 : Fcn  Expr=u(1)*(u(2)>0)
  Fcn4 : Fcn  Expr=u(1)*(u(2)<=u(3))
  Fcn5 : Fcn  Expr=u(1)*(u(2)>u(3))
  Fcn6 : Fcn  Expr=-1*(u(1)-1)^2/w^2
  Gain1 : Gain  Gain=1.5
  Gain2 : Gain
  Gain24 : Gain  Gain=1.28
  Gain25 : Gain  Gain=4
  Gain26 : Gain  Gain=lopt
  Gain27 : Gain  Gain=1059.7
  Gain28 : Gain  Gain=1.5
  Gain3 : Gain  Gain=lopt
  Gain4 : Gain  Gain=lopt
  Math Function : Math  SaturateOnIntegerOverflow=on
  Mux : Mux  Inputs=2
  Mux1 : Mux  Inputs=2
  Mux2 : Mux  Inputs=2
  Mux3 : Mux  Inputs=3
  Mux4 : Mux  Inputs=3
  Percent Fast Twitch : Constant  Value=FT
  Sum : Sum  Inputs=|++
  Sum1 : Sum  Inputs=+|+
  Sum2 : Sum  Inputs=-|-
  Sum3 : Sum  Inputs=+|+
  Sum4 : Sum  Inputs=++-
  Sum5 : Sum  Inputs=++-
  Sum6 : Sum
  Sum7 : Sum
  Terminator : Terminator
  Terminator1 : Terminator
  Power : Outport
  wires:
  [m] -> Divide12/2
  [fce] -> Divide7/1
  [act] -> Mux/2
  [stim] -> Mux/1
  Gain26/1 -> Gain27/1
  Gain24/1 -> Sum/1
  Divide10/1 -> Sum6/1
  Divide9/1 -> Sum5/3
  Sum4/1 -> Mux3/1
  Divide12/1 -> Power/1  "power"
  Fcn4/1 -> Sum7/1
  [Fiso] -> Divide8/1
  Fcn6/1 -> Math Function/1
  [A] -> Divide5/3
  [ham_dot] -> Divide11/1
  Divide11/1 -> Sum6/2
  [m] -> Divide9/3
  [lce_norm] -> Mux4/2
  [ham_dot] -> Divide10/1
  Sum5/1 -> Mux4/1
  Sum6/1 -> Sum5/1
  [SHORT] -> Sum4/2
  Constant19/1 -> Mux3/3
  Mux4/1 -> Fcn5/1
  Fcn5/1 -> Sum7/2
  [vce_norm] -> Divide5/2
  [a_l] -> Gain1/1
  [Aam] -> Divide6/2
  Gain1/1 -> Divide5/1
  Constant16/1 -> Divide2/3
  Constant17/1 -> Divide3/3
  [Fiso] -> Divide11/3
  [vce_norm] -> Gain4/1
  Divide3/1 -> Sum2/1
  Gain25/1 -> [a_l]  "a_l"
  Math Function/1 -> [Fiso]
  "Aam "/1 -> [Aam]
  Constant10/1 -> Divide1/2  "VCEft"
  Divide2/1 -> Sum2/2
  [vce_norm] -> Divide2/2
  Divide1/1 -> Divide3/1  "a_ft"
  [vce_norm] -> Mux1/2
  Sum7/1 -> Divide12/1
  Fcn3/1 -> Sum3/2
  Constant22/1 -> Mux4/3
  Divide5/1 -> Mux2/1
  Constant14/1 -> Divide/1
  Divide6/1 -> Sum4/1
  Divide/1 -> Gain25/1, Divide2/1  "a_st"
  [ham_dot] -> Divide6/1
  Sum1/1 -> "Aam "/1, As/1, [A]  "A"
  Constant18/1 -> Divide6/3
  Constant15/1 -> Divide1/1
  Divide4/1 -> Mux1/1
  Mux1/1 -> Fcn2/1
  [vce_norm] -> Divide3/2
  Fcn1/1 -> Sum1/2
  Fcn/1 -> Sum1/1
  [vce_norm] -> Gain3/1
  Divide7/1 -> Sum4/3
  Constant13/1 -> Sum/2
  Divide8/1 -> Sum5/2
  As/1 -> [As]
  Constant20/1 -> Divide10/2
  Sum2/1 -> Divide4/1
  [m] -> Divide7/3
  [fce] -> Divide9/1
  Sum/1 -> [ham_dot]  "Ham_dot"
  Mux/1 -> Fcn1/1, Fcn/1
  Percent Fast Twitch/1 -> Gain24/1
  [vce_norm] -> Mux2/2
  Constant21/1 -> Divide11/2
  Constant2/1 -> Gain26/1  "PCSAL"
  [SHORT] -> Divide8/2
  Mux3/1 -> Fcn4/1
  [lce_norm] -> Mux3/2
  Gain28/1 -> Divide4/2
  Constant9/1 -> Divide/2  "VCEst"
  Gain27/1 -> [m]  "Mass"
  Mux2/1 -> Fcn3/1
  Sum3/1 -> [SHORT]
  Fcn2/1 -> Sum3/1
  [As] -> Gain28/1
  Dynamics/1 -> Demux/1
  Stimulation/1 -> [stim]
  Demux/1 -> [fce]
  Demux/2 -> [lce_norm]  "lce [lopt]"
  Demux/3 -> [vce_norm]  "vce [lopt]"
  Demux/5 -> [act]
  Demux/4 -> Terminator/1
  [lce_norm] -> Gain2/1
  Gain2/1 -> Fcn6/1
  Demux/6 -> Terminator1/1
  Gain3/1 -> Divide9/2
  Gain4/1 -> Divide7/2

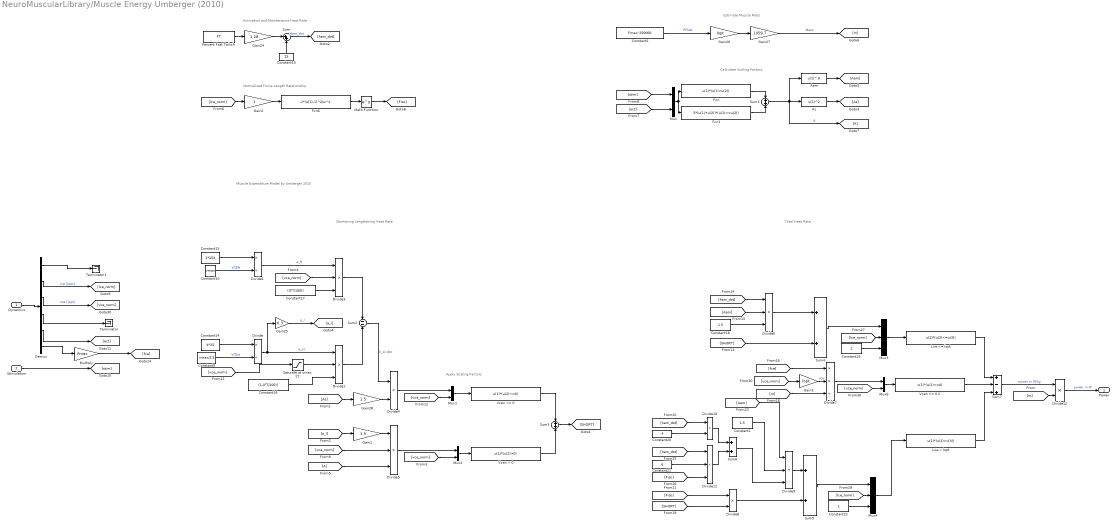
== system NeuroMuscularLibrary/Muscle Energy Umberger (2010) ==
  note: Activation and Maintenance Heat Rate
  note: Normalized Force-Length Relationship
  note: Shortening Lengthening Heat Rate
  note: Apply Scaling Factors
  note: Calculate Scaling Factors
  note: Estimate Muscle Mass
  note: Total Heat Rate
  note: Muscle Expenditure Model by Umberger 2010
  Dynamics : Inport
  Stimulation : Inport  Port=2
  "Aam " : Fcn  Expr=u(1)^.6
  As : Fcn  Expr=u(1)^2
  Constant1 : Constant  Value=1.5
  Constant10 : Constant  Value=vmax
  Constant13 : Constant  Value=25
  Constant14 : Constant  Value=4*25
  Constant15 : Constant  Value=1*153
  Constant16 : Constant  Value=(1-(FT/100))
  Constant17 : Constant  Value=((FT/100))
  Constant18 : Constant  Value=1.5
  Constant19 : Constant
  Constant2 : Constant  Value=Fmax/ 250000
  Constant20 : Constant  Value=.4
  Constant21 : Constant  Value=.6
  Constant22 : Constant
  Constant9 : Constant  Value=vmax/2.5
  Demux : Demux  Outputs=6
  Divide : Product  Inputs=*/
  Divide1 : Product  Inputs=*/
  Divide{4,8,10,12} (4 alike) : Product  Inputs=**
  Divide{2..3,5..6,9,11} (6 alike) : Product  Inputs=***
  Divide7 : Product  Inputs=**/
  Fcn : Fcn  Expr=u(1)*(u(1)>u(2))
  Fcn1 : Fcn  Expr=.5*(u(1)+u(2))*(u(1)<=u(2))
  Fcn6 : Fcn  Expr=-1*(u(1)-1)^2/w^2
  Gain1 : Gain  Gain=1.5
  Gain2 : Gain
  Gain24 : Gain  Gain=1.28
  Gain25 : Gain  Gain=0.3
  Gain26 : Gain  Gain=lopt
  Gain27 : Gain  Gain=1059.7
  Gain28 : Gain  Gain=1.5
  Gain3 : Gain  Gain=lopt
  Lce <= lopt : Fcn  Expr=u(1)*(u(2)<=u(3))
  Lce > lopt : Fcn  Expr=u(1)*(u(2)>u(3))
  Math Function : Math  SaturateOnIntegerOverflow=on
  Multiply : Gain  Gain=Fmax
  Mux{,1..2,6} (4 alike) : Mux  Inputs=2
  Mux3 : Mux  Inputs=3
  Mux4 : Mux  Inputs=3
  Percent Fast Twitch : Constant  Value=FT
  Saturate at vmax ST : Saturate  UpperLimit=vmax/2.5  LowerLimit=-vmax/2.5  ZeroCross=off
  Sum : Sum  Inputs=|++
  Sum1 : Sum  Inputs=+|+
  Sum2 : Sum  Inputs=-|-
  Sum3 : Sum  Inputs=+|+
  Sum4 : Sum
  Sum5 : Sum
  Sum6 : Sum
  Sum7 : Sum  Inputs=+-+
  Terminator : Terminator
  Terminator1 : Terminator
  "Vcen <= 0 " : Fcn  Expr=u(1)*(u(2)<=0)
  Vcen <= 0 2 : Fcn  Expr=u(1)*(u(2)<=0)
  Vcen > 0 : Fcn  Expr=u(1)*(u(2)>0)
  Power : Outport
  wires:
  Lce > lopt/1 -> Sum7/3
  Lce <= lopt/1 -> Sum7/1
  Multiply/1 -> [fce]
  Saturate at vmax ST/1 -> Divide2/2
  [m] -> Divide12/2
  Divide9/1 -> Sum5/1
  [Aam] -> Divide9/1
  Constant1/1 -> Divide9/2
  [m] -> Divide7/3
  [fce] -> Divide7/1
  [vce_norm] -> Gain3/1
  [act] -> Mux/2
  [stim] -> Mux/1
  Gain26/1 -> Gain27/1
  Gain24/1 -> Sum/1
  Divide10/1 -> Sum6/1
  Sum4/1 -> Mux3/1
  Divide12/1 -> Power/1  "power in W"
  [Fiso] -> Divide8/1
  Fcn6/1 -> Math Function/1
  [A] -> Divide5/3
  [ham_dot] -> Divide11/1
  Divide11/1 -> Sum6/2
  [lce_norm] -> Mux4/2
  [ham_dot] -> Divide10/1
  Sum5/1 -> Mux4/1
  Sum6/1 -> Divide9/3
  [SHORT] -> Sum4/2
  Constant19/1 -> Mux3/3
  Mux4/1 -> Lce > lopt/1
  [vce_norm] -> Divide5/2
  [a_l] -> Gain1/1
  [Aam] -> Divide6/2
  Gain1/1 -> Divide5/1
  Constant16/1 -> Divide2/3
  Constant17/1 -> Divide3/3
  [Fiso] -> Divide11/3
  Divide3/1 -> Sum2/1
  Gain25/1 -> [a_l]  "a_l"
  Math Function/1 -> [Fiso]
  "Aam "/1 -> [Aam]
  Constant10/1 -> Divide1/2  "VCEft"
  Divide2/1 -> Sum2/2
  [vce_norm] -> Saturate at vmax ST/1
  Divide1/1 -> Divide3/1  "a_ft"
  [vce_norm] -> Mux1/2
  Sum7/1 -> Divide12/1  "power in W/kg"
  Vcen > 0/1 -> Sum3/2
  Constant22/1 -> Mux4/3
  Divide5/1 -> Mux2/1
  Constant14/1 -> Divide/1
  Divide6/1 -> Sum4/1
  Divide/1 -> Gain25/1, Divide2/1  "a_st"
  [ham_dot] -> Divide6/1
  Sum1/1 -> "Aam "/1, As/1, [A]  "A"
  Constant18/1 -> Divide6/3
  Constant15/1 -> Divide1/1
  Divide4/1 -> Mux1/1
  Mux1/1 -> "Vcen <= 0 "/1
  [vce_norm] -> Divide3/2
  Fcn1/1 -> Sum1/2
  Fcn/1 -> Sum1/1
  Constant13/1 -> Sum/2
  Divide8/1 -> Sum5/2
  As/1 -> [As]
  Constant20/1 -> Divide10/2
  Sum2/1 -> Divide4/1  "h_sl dot"
  Sum/1 -> [ham_dot]  "Ham_dot"
  Mux/1 -> Fcn1/1, Fcn/1
  Percent Fast Twitch/1 -> Gain24/1
  [vce_norm] -> Mux2/2
  Constant21/1 -> Divide11/2
  Constant2/1 -> Gain26/1  "PCSAL"
  [SHORT] -> Divide8/2
  Mux3/1 -> Lce <= lopt/1
  [lce_norm] -> Mux3/2
  Gain28/1 -> Divide4/2
  Constant9/1 -> Divide/2  "VCEst"
  Gain27/1 -> [m]  "Mass"
  Mux2/1 -> Vcen > 0/1
  Sum3/1 -> [SHORT]
  "Vcen <= 0 "/1 -> Sum3/1
  [As] -> Gain28/1
  Dynamics/1 -> Demux/1
  Stimulation/1 -> [stim]
  Demux/1 -> Terminator1/1
  Demux/2 -> [lce_norm]  "lce [lopt]"
  Demux/3 -> [vce_norm]  "vce [lopt]"
  Demux/5 -> [act]
  Demux/4 -> Terminator/1
  [lce_norm] -> Gain2/1
  Gain2/1 -> Fcn6/1
  Demux/6 -> Multiply/1
  [vce_norm] -> Mux6/2
  Divide7/1 -> Mux6/1
  Mux6/1 -> Vcen <= 0 2/1
  Vcen <= 0 2/1 -> Sum7/2
  Gain3/1 -> Divide7/2  "vce"
